simulink model "insulin_glucose"  (R2023a)
settings: Solver=VariableStepAuto  StartTime=0.0  StopTime=10  RelTol=1e-3
libraries: simulink x2
settings Model: Creator=User  LastModifiedBy=User
settings OptimizationCC: ReuseModelBlockBuffer=off
settings DebuggingCC: UnconnectedInputMsg=warning  UnconnectedOutputMsg=warning  UnconnectedLineMsg=warning
settings ModelReferenceCC: EnableRefExpFcnMdlSchedulingChecks=on
settings RTWCC: DLArmComputeVersion=19.05

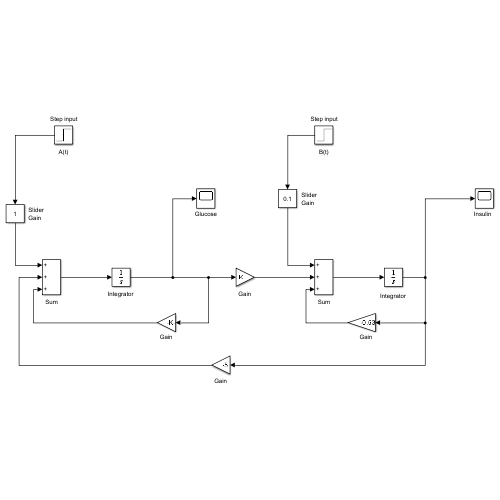
[thumbnail: Simulink's stored preview of the top-level diagram]
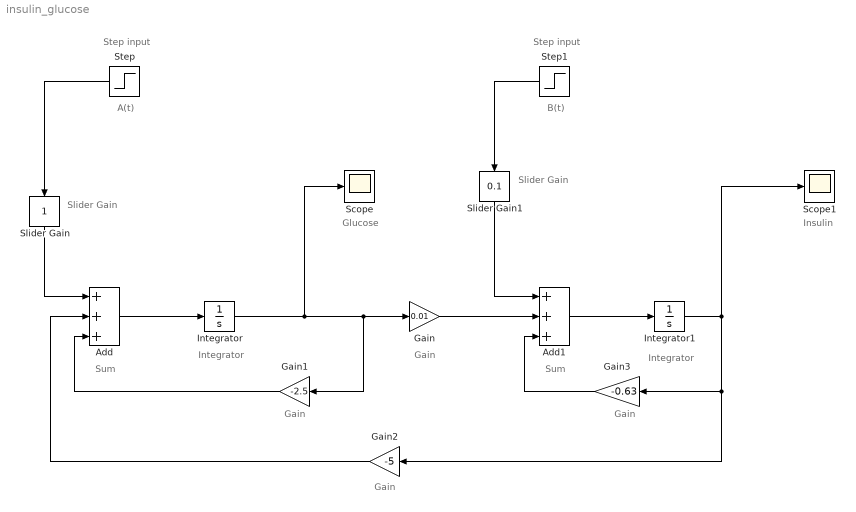
== system insulin_glucose ==
  note: Step input
  note: A(t)
  note: Slider
      | Gain
  note: Gain
  note: Insulin
  note: Slider
      | Gain
  note: Sum
  note: Step input
  note: Integrator
  note: Sum
  note: B(t)
  note: Integrator
  note: Gain
  note: Gain
  note: Glucose
  note: Gain
  Add : Sum  Inputs=+++
  Add1 : Sum  Inputs=+++
  Gain : Gain  Gain=0.01
  Gain1 : Gain  Gain=-2.5
  Gain2 : Gain  Gain=-5
  Gain3 : Gain  Gain=-0.63
  Integrator : Integrator
  Integrator1 : Integrator
  Scope : Scope
  Scope1 : Scope
  Slider Gain : simulink/Math Operations/Slider Gain  gain=1  low=0  high=2
  Slider Gain1 : simulink/Math Operations/Slider Gain  gain=0.1  low=0  high=2
  Step : Step  Before=1  SampleTime=0
  Step1 : Step  After=0  SampleTime=0
  wires:
  Gain3/1 -> Add1/3
  Step/1 -> Slider Gain/1
  Integrator1/1 -> Gain3/1, Gain2/1, Scope1/1
  Slider Gain1/1 -> Add1/1
  Gain1/1 -> Add/3
  Step1/1 -> Slider Gain1/1
  Add1/1 -> Integrator1/1
  Gain2/1 -> Add/2
  Integrator/1 -> Scope/1, Gain1/1, Gain/1
  Gain/1 -> Add1/2
  Add/1 -> Integrator/1
  Slider Gain/1 -> Add/1
